simulink model "can_msg_m250"  (Simulink 8.4)
settings: Solver=FixedStepDiscrete  StartTime=0.0  StopTime=inf  RelTol=1e-3
PreLoadFcn:
  | openecu_make_rtw_hook('model_load', 'can_msg_m250')
PostLoadFcn:
  | openecu_make_rtw_hook('model_loaded', 'can_msg_m250')
InitFcn:
  | openecu_make_rtw_hook('model_init', 'can_msg_m250')
undefined symbols (not defined in the file): adic_vset, Brake, Grade, PRND, T_Req
libraries: pcx x4, simulink x1, pcp_CCP_Configuration x1, prtw x1, put x1
settings Model: Creator=jtough  LastModifiedBy=Administrator  TunableVars=adic_vactual,adic_vset  TunableVarsStorageClass=ExportedGlobal,ExportedGlobal  TunableVarsTypeQualifier=OE_CAL,OE_CAL
settings ConfigSet: Description=|
  | OpenECU configuration set for code generation under RTW (RSIM).
  | --
  | OpenECU RTW (RSIM) support is deprecated, please use the OpenECU RTW (RTMODEL) configuration set.
settings SolverCC: PositivePriorityOrder=on
settings OptimizationCC: InlineParams=on  InlineInvariantSignals=on  FoldNonRolledExpr=off
settings DebuggingCC: SaveWithParameterizedLinksMsg=none  SolverPrmCheckMsg=none  MultiTaskDSMMsg=warning  MultiTaskCondExecSysMsg=none  SingleTaskRateTransMsg=error  CheckMatrixSingularityMsg=warning  VectorMatrixConversionMsg=warning  SignalLabelMismatchMsg=warning
settings HardwareCC: ProdLargestAtomicInteger=Long  ProdLargestAtomicFloat=Double  ProdIntDivRoundTo=Zero  ProdEndianess=BigEndian  ProdHWDeviceType=Freescale->32-bit PowerPC  TargetLargestAtomicInteger=Long  TargetLargestAtomicFloat=Double  TargetIntDivRoundTo=Zero  TargetEndianess=BigEndian  TargetHWDeviceType=Freescale->32-bit PowerPC  ProdEqTarget=off
settings RTWCC: SystemTargetFile=openecu.tlc  TemplateMakefile=openecu_r2014b_64.tmf  Description=OpenECU Platform Target (GRT, RSIM based)  RetainRTWFile=on  ProcessScript=openecu_make_rtw_hook  IncludeERTFirstTime=on
settings STFCustomTargetCC: TargetLibSuffix=.a  ModelReferenceCompliant=off  GeneratePreprocessorConditionals=Disable all  MATLABClassNameForMDSCustomization=Simulink.SoftwareTarget.TargetSpecificTriggerConfigurationBase  SystemTargetFile=openecu.tlc
settings RSimTargetCC: TargetLibSuffix=.a  ERTMultiwordTypeDef=System defined  ERTMultiwordLength=256  ModelReferenceCompliant=off  ParMdlRefBuildCompliant=off  CompOptLevelCompliant=off  ConcurrentExecutionCompliant=off  MatFileLogging=off  EnableShiftOperators=on
settings EnumStrPairs: String=prefix_name

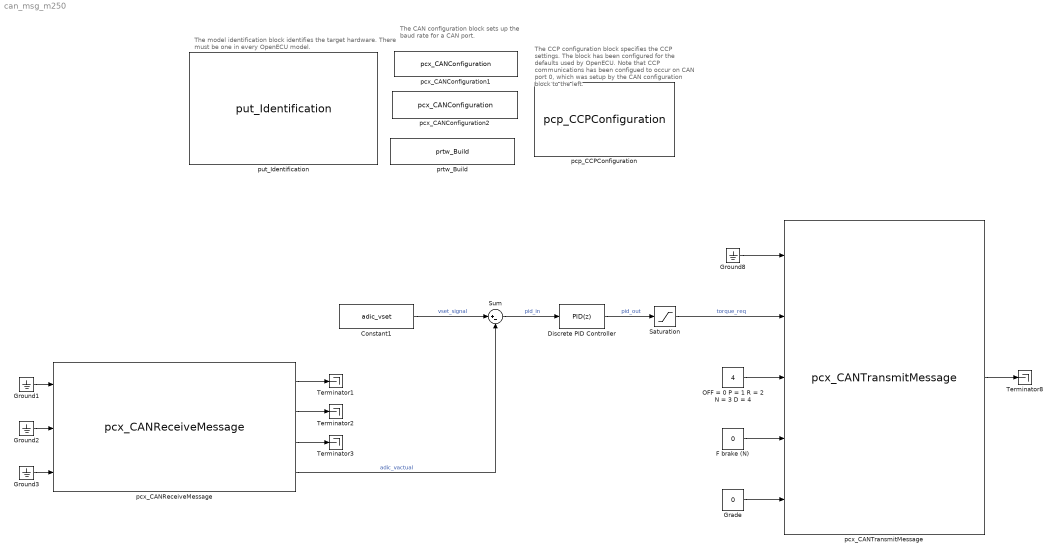
== system can_msg_m250 ==
  note: The model identification block identifies the target hardware.
      | There must be one in every OpenECU model.
  note: The CAN configuration block sets up
      | the baud rate for a CAN port.
  note: The CCP configuration block specifies the CCP
      | settings. The block has been configured for the
      | defaults used by OpenECU. Note that CCP
      | communications has been configued to occur
      | on CAN port 0, which was setup by the CAN
      | configuration block to the left.
  Constant1 : Constant  Value=adic_vset  OutDataTypeStr=single
  Discrete PID Controller : simulink/Continuous/PID Controller  Controller=PID  TimeDomain=Discrete-time  SampleTime=0.01  IntegratorMethod=Forward Euler  FilterMethod=Forward Euler  Form=Parallel  P=25.424578918926  I=2.59319385779654  D=2.72020870275003  N=42.8816743973314  InitialConditionSource=internal  InitialConditionForIntegrator=0  InitialConditionForFilter=0  ExternalReset=none  LimitOutput=on  UpperSaturationLimit=290  LowerSaturationLimit=-290  LinearizeAsGain=off  AntiWindupMode=none  Kb=1  TrackingMode=off  Kt=1  PParamMin=[]  PParamMax=[]  IParamMin=[]  IParamMax=[]  DParamMin=[]  DParamMax=[]  NParamMin=[]  NParamMax=[]  KbParamMin=[]  KbParamMax=[]  KtParamMin=[]  KtParamMax=[]  POutMin=[]  POutMax=[]  IOutMin=[]  IOutMax=[]  DOutMin=[]  DOutMax=[]  NOutMin=[]  NOutMax=[]  KbOutMin=[]  KbOutMax=[]  KtOutMin=[]  KtOutMax=[]  IntegratorOutMin=[]  IntegratorOutMax=[]  FilterOutMin=[]  FilterOutMax=[]  SumOutMin=[]  SumOutMax=[]  SumI1OutMin=[]  SumI1OutMax=[]  SumI2OutMin=[]  SumI2OutMax=[]  SumI3OutMin=[]  SumI3OutMax=[]  SumDOutMin=[]  SumDOutMax=[]  SaturationOutMin=[]  SaturationOutMax=[]  IntegratorContinuousStateAttributes=''  IntegratorStateMustResolveToSignalObject=off  IntegratorRTWStateStorageClass=Auto  FilterContinuousStateAttributes=''  FilterStateMustResolveToSignalObject=off  FilterRTWStateStorageClass=Auto  DifferentiatorICPrevScaledInput=0  DifferentiatorOutMin=[]  DifferentiatorOutMax=[]  UseFilter=off
  F brake (N) : Constant  Value=0  OutDataTypeStr=single
  Grade : Constant  Value=0  OutDataTypeStr=single
  Ground{1..3,8} (4 alike) : Ground
  OFF = 0 P = 1 R = 2 N = 3 D = 4 : Constant  Value=4  OutDataTypeStr=single
  Saturation : Saturate  UpperLimit=255  LowerLimit=-255
  Sum : Sum  Inputs=|+-
  Terminator{1..3,8} (4 alike) : Terminator
  pcp_CCPConfiguration : pcp_CCP_Configuration/pcp_CCPConfiguration  pcpl_rx_msgid=1785  pcpl_tx_msgid=1784  pcpl_station_id=0  bus_id=CAN 0 (pin A28+A43)  pcpl_ccpenabled=on  pcpl_rx_ext_id=off  pcpl_tx_ext_id=off  pcpl_caltool=Generic
  pcx_CANConfiguration1 : pcx/pcx_CANConfiguration  bit_rate=1000 kBps  bus_id=CAN 0 (pin A28+A43)
  pcx_CANConfiguration2 : pcx/pcx_CANConfiguration  bit_rate=1000 kBps  bus_id=CAN 1 (pin A29+A44)
  pcx_CANReceiveMessage : pcx/pcx_CANReceiveMessage  pcxl_msg_id=257  pcxl_msg_length=8  pcxl_field_start_pos=[0]  pcxl_field_width=[8]  pcxl_field_is_signed=[0]  pcxl_type_codes=[0]  pcxl_field_mnemonics=<v (km/h)>  bus_id=CAN 0 (pin A28+A43)  pcxl_sample_time=0.01  pcxl_use_extended_ids=off  pcxl_provide_timestamp=off  pcxl_provide_sim_inputs=off
  pcx_CANTransmitMessage : pcx/pcx_CANTransmitMessage  pcxl_msg_id=1025  pcxl_msg_length=8  pcxl_field_start_pos=[0,8,16,24]  pcxl_field_width=[8,8,8,8]  pcxl_field_is_signed=[0,0,0,0]  pcxl_type_codes=[0,0,0,0]  pcxl_field_mnemonics=T_Req,PRND,Brake,Grade  bus_id=CAN 0 (pin A28+A43)  pcxl_use_extended_ids=off  pcxl_provide_status=off  pcxl_provide_sim_outputs=off
  prtw_Build : prtw/prtw_Build
  put_Identification : put/put_Identification  put_id_marque=M250  dummy_marque_00=01T-068883-000  dummy_marque_01=01T-068432-000  dummy_marque_02=01T-068696-000  dummy_marque_03=01T-068276-000  dummy_marque_04=01T-068144-000  dummy_marque_05=01T-068148-000  dummy_marque_06=01T-068787-000  dummy_marque_07=01T-068408-000  dummy_marque_08=01T-063522-000  dummy_marque_09=01T-063512-000  dummy_marque_10=01T-063522-000  put_id_part_number=01T-068276-000  put_id_num_marques=7  put_id_max_marques=11  put_id_issue_number=3  put_id_min_issue_num=2  put_id_naming=Generic pin naming  put_id_name=Application name here  put_id_description=Description here  put_id_major_ver_str=1  put_id_major_ver_num=1  put_id_minor_ver_str=0  put_id_minor_ver_num=0  put_id_subminor_ver_str=0  put_id_subminor_ver_num=0  put_id_copyright=(none)  put_id_target=Unused  put_id_target_type=M250  put_id_subtype=000  put_id_family=Unused  put_id_variant=Unused  put_id_A450_variant=0  put_id_G400_variant=0  put_id_G800_variant=0  put_id_G850_variant=Unused  put_id_M001_variant=0  put_id_M250_variant=Unused  put_id_M460_variant=Unused  put_id_M461_variant=Unused  put_id_U082_variant=Unused  put_id_U82_variant=Unused
  wires:
  pcx_CANTransmitMessage/1 -> Terminator8/1
  Ground8/1 -> pcx_CANTransmitMessage/1
  Discrete PID Controller/1 -> Saturation/1  "pid_out"
  OFF = 0 P = 1 R = 2 N = 3 D = 4/1 -> pcx_CANTransmitMessage/3
  F brake (N)/1 -> pcx_CANTransmitMessage/4
  Sum/1 -> Discrete PID Controller/1  "pid_in"
  pcx_CANReceiveMessage/3 -> Terminator3/1
  pcx_CANReceiveMessage/2 -> Terminator2/1
  pcx_CANReceiveMessage/1 -> Terminator1/1
  Ground1/1 -> pcx_CANReceiveMessage/1
  Ground2/1 -> pcx_CANReceiveMessage/2
  Ground3/1 -> pcx_CANReceiveMessage/3
  Constant1/1 -> Sum/1  "vset_signal"
  Grade/1 -> pcx_CANTransmitMessage/5
  Saturation/1 -> pcx_CANTransmitMessage/2  "torque_req"
  pcx_CANReceiveMessage/4 -> Sum/2  "adic_vactual"
